simulink library "halout"  (R2021b)
settings: Solver=VariableStepAuto  StartTime=0.0  StopTime=10.0  RelTol=1e-3
undefined symbols (not defined in the file): C_TASK_5MS_S, FALSE, KHAL_CAN1FDAPS3E2E_flg, KHAL_CAN1FDAPS3TxReq_flg, KHAL_CAN1FDVCU2E2E_flg, KHAL_CAN1FDVCU2TxReq_flg, KHAL_CAN1FDVCU3E2E_flg, KHAL_CAN1FDVCU3TxReq_flg, KHAL_CAN1TxReq_flg, KHAL_CAN2TxReq_flg, KHAL_CAN3FDVCU1TxReq_flg, KHAL_CAN3FDVCU2E2E_flg, KHAL_CAN3FDVCU2TxReq_flg, KHAL_CAN3TxReq_flg, KHAL_CAN4FDVCU1E2E_flg, KHAL_CAN4FDVCU1TxReq_flg, KHAL_CAN4TxReq_flg, KHAL_CAN5TxReq_flg, ONE_INT, TRUE, ZERO_INT
libraries: FVT_lib x383, simulink x179
(part 18 of 20)

== system halout/HAL_OUT/CAN4/FD_THCM2_0x186/FDEXV2Cmd ==
  FDEXV2Cmd : Inport
  Data Type Conversion : DataTypeConversion  OutDataTypeStr=uint16  RndMeth=Round
  CAN4_FD_EXV2_Cmd : Outport
  wires:
  Data Type Conversion/1 -> CAN4_FD_EXV2_Cmd/1
  FDEXV2Cmd/1 -> Data Type Conversion/1

== system halout/HAL_OUT/CAN4/FD_THCM2_0x186/FDFWVCmd ==
  FDFWVCmd : Inport
  Data Type Conversion : DataTypeConversion  OutDataTypeStr=uint8  RndMeth=Round
  CAN4_FD_FWV_Cmd : Outport
  wires:
  Data Type Conversion/1 -> CAN4_FD_FWV_Cmd/1
  FDFWVCmd/1 -> Data Type Conversion/1

== system halout/HAL_OUT/CAN4/FD_THCM2_0x186/FDFrLeAPTCHeatPwrCmd ==
  FDFrLeAPTCHeatPwrCmd : Inport
  Data Type Conversion : DataTypeConversion  OutDataTypeStr=uint8  RndMeth=Round
  convert_out : FVT_lib/hal/convert_out  gain=25  offset=0
  CAN4_FD_FrLeAPTCHeatPwr_Cmd : Outport
  wires:
  Data Type Conversion/1 -> CAN4_FD_FrLeAPTCHeatPwr_Cmd/1
  convert_out/1 -> Data Type Conversion/1
  FDFrLeAPTCHeatPwrCmd/1 -> convert_out/1

== system halout/HAL_OUT/CAN4/FD_THCM2_0x186/FDFrRiAPTCHeatPwrCmd ==
  FDFrRiAPTCHeatPwrCmd : Inport
  Data Type Conversion : DataTypeConversion  OutDataTypeStr=uint8  RndMeth=Round
  convert_out : FVT_lib/hal/convert_out  gain=25  offset=0
  CAN4_FD_FrRiAPTCHeatPwr_Cmd : Outport
  wires:
  Data Type Conversion/1 -> CAN4_FD_FrRiAPTCHeatPwr_Cmd/1
  convert_out/1 -> Data Type Conversion/1
  FDFrRiAPTCHeatPwrCmd/1 -> convert_out/1

== system halout/HAL_OUT/CAN4/FD_THCM2_0x186/FDFrWPTCHeatPwrCmd ==
  FDFrWPTCHeatPwrCmd : Inport
  Data Type Conversion : DataTypeConversion  OutDataTypeStr=uint16  RndMeth=Round
  CAN4_FD_FrWPTCHeatPwr_Cmd : Outport
  wires:
  Data Type Conversion/1 -> CAN4_FD_FrWPTCHeatPwr_Cmd/1
  FDFrWPTCHeatPwrCmd/1 -> Data Type Conversion/1

== system halout/HAL_OUT/CAN4/FD_THCM2_0x186/FDRrAPTCHeatPwrCmd ==
  FDRrAPTCHeatPwrCmd : Inport
  Data Type Conversion : DataTypeConversion  OutDataTypeStr=uint8  RndMeth=Round
  convert_out : FVT_lib/hal/convert_out  gain=25  offset=0
  CAN4_FD_RrAPTCHeatPwr_Cmd : Outport
  wires:
  Data Type Conversion/1 -> CAN4_FD_RrAPTCHeatPwr_Cmd/1
  convert_out/1 -> Data Type Conversion/1
  FDRrAPTCHeatPwrCmd/1 -> convert_out/1

== system halout/HAL_OUT/CAN4/FD_THCM2_0x186/FDSOTXVCmd ==
  FDSOTXVCmd : Inport
  Data Type Conversion : DataTypeConversion  OutDataTypeStr=uint8  RndMeth=Round
  CAN4_FD_SOTXV_Cmd : Outport
  wires:
  Data Type Conversion/1 -> CAN4_FD_SOTXV_Cmd/1
  FDSOTXVCmd/1 -> Data Type Conversion/1

== system halout/HAL_OUT/CAN4/FD_THCM2_0x186/FDSOV1Cmd ==
  FDSOV1Cmd : Inport
  Data Type Conversion : DataTypeConversion  OutDataTypeStr=uint8  RndMeth=Round
  CAN4_FD_SOV1_Cmd : Outport
  wires:
  Data Type Conversion/1 -> CAN4_FD_SOV1_Cmd/1
  FDSOV1Cmd/1 -> Data Type Conversion/1

== system halout/HAL_OUT/CAN4/FD_THCM2_0x186/FDSOV2Cmd ==
  FDSOV2Cmd : Inport
  Data Type Conversion : DataTypeConversion  OutDataTypeStr=uint8  RndMeth=Round
  CAN4_FD_SOV2_Cmd : Outport
  wires:
  Data Type Conversion/1 -> CAN4_FD_SOV2_Cmd/1
  FDSOV2Cmd/1 -> Data Type Conversion/1

== system halout/HAL_OUT/CAN4/FD_THCM2_0x186/FDSOV3Cmd ==
  FDSOV3Cmd : Inport
  Data Type Conversion : DataTypeConversion  OutDataTypeStr=uint8  RndMeth=Round
  CAN4_FD_SOV3_Cmd : Outport
  wires:
  Data Type Conversion/1 -> CAN4_FD_SOV3_Cmd/1
  FDSOV3Cmd/1 -> Data Type Conversion/1

== system halout/HAL_OUT/CAN4/FD_THCM2_0x186/FDTWVCmd ==
  FDTWVCmd : Inport
  Data Type Conversion : DataTypeConversion  OutDataTypeStr=uint8  RndMeth=Round
  convert_out : FVT_lib/hal/convert_out  gain=0.392  offset=0
  CAN4_FD_TWV_Cmd : Outport
  wires:
  Data Type Conversion/1 -> CAN4_FD_TWV_Cmd/1
  convert_out/1 -> Data Type Conversion/1
  FDTWVCmd/1 -> convert_out/1

== system halout/HAL_OUT/CAN4/FD_VCU1_0x116/AllDoorSW ==
  AllDoorSW : Inport
  Data Type Conversion : DataTypeConversion  OutDataTypeStr=uint8  RndMeth=Round
  CAN4_AllDoorSW : Outport
  wires:
  Data Type Conversion/1 -> CAN4_AllDoorSW/1
  AllDoorSW/1 -> Data Type Conversion/1

== system halout/HAL_OUT/CAN4/FD_VCU1_0x116/AmbLightBreath1 ==
  AmbLightBreath1 : Inport
  Data Type Conversion : DataTypeConversion  OutDataTypeStr=uint8  RndMeth=Round
  CAN4_AmbLightBreath1 : Outport
  wires:
  Data Type Conversion/1 -> CAN4_AmbLightBreath1/1
  AmbLightBreath1/1 -> Data Type Conversion/1

== system halout/HAL_OUT/CAN4/FD_VCU1_0x116/AmbLightBreath2 ==
  AmbLightBreath2 : Inport
  Data Type Conversion : DataTypeConversion  OutDataTypeStr=uint8  RndMeth=Round
  CAN4_AmbLightBreath2 : Outport
  wires:
  Data Type Conversion/1 -> CAN4_AmbLightBreath2/1
  AmbLightBreath2/1 -> Data Type Conversion/1

== system halout/HAL_OUT/CAN4/FD_VCU1_0x116/AmbLightBreath3 ==
  AmbLightBreath3 : Inport
  Data Type Conversion : DataTypeConversion  OutDataTypeStr=uint8  RndMeth=Round
  CAN4_AmbLightBreath3 : Outport
  wires:
  Data Type Conversion/1 -> CAN4_AmbLightBreath3/1
  AmbLightBreath3/1 -> Data Type Conversion/1

== system halout/HAL_OUT/CAN4/FD_VCU1_0x116/AmbLightBrightness1 ==
  AmbLightBrightness1 : Inport
  Data Type Conversion : DataTypeConversion  OutDataTypeStr=uint8  RndMeth=Round
  CAN4_AmbLightBrightness1 : Outport
  wires:
  Data Type Conversion/1 -> CAN4_AmbLightBrightness1/1
  AmbLightBrightness1/1 -> Data Type Conversion/1

== system halout/HAL_OUT/CAN4/FD_VCU1_0x116/AmbLightBrightness2 ==
  AmbLightBrightness2 : Inport
  Data Type Conversion : DataTypeConversion  OutDataTypeStr=uint8  RndMeth=Round
  CAN4_AmbLightBrightness2 : Outport
  wires:
  Data Type Conversion/1 -> CAN4_AmbLightBrightness2/1
  AmbLightBrightness2/1 -> Data Type Conversion/1

== system halout/HAL_OUT/CAN4/FD_VCU1_0x116/AmbLightBrightness3 ==
  AmbLightBrightness3 : Inport
  Data Type Conversion : DataTypeConversion  OutDataTypeStr=uint8  RndMeth=Round
  CAN4_AmbLightBrightness3 : Outport
  wires:
  Data Type Conversion/1 -> CAN4_AmbLightBrightness3/1
  AmbLightBrightness3/1 -> Data Type Conversion/1

== system halout/HAL_OUT/CAN4/FD_VCU1_0x116/AmbLightColor1 ==
  AmbLightColor1 : Inport
  Data Type Conversion : DataTypeConversion  OutDataTypeStr=uint8  RndMeth=Round
  CAN4_AmbLightColor1 : Outport
  wires:
  Data Type Conversion/1 -> CAN4_AmbLightColor1/1
  AmbLightColor1/1 -> Data Type Conversion/1

== system halout/HAL_OUT/CAN4/FD_VCU1_0x116/AmbLightColor2 ==
  AmbLightColor2 : Inport
  Data Type Conversion : DataTypeConversion  OutDataTypeStr=uint8  RndMeth=Round
  CAN4_AmbLightColor2 : Outport
  wires:
  Data Type Conversion/1 -> CAN4_AmbLightColor2/1
  AmbLightColor2/1 -> Data Type Conversion/1

== system halout/HAL_OUT/CAN4/FD_VCU1_0x116/AmbLightColor3 ==
  AmbLightColor3 : Inport
  Data Type Conversion : DataTypeConversion  OutDataTypeStr=uint8  RndMeth=Round
  CAN4_AmbLightColor3 : Outport
  wires:
  Data Type Conversion/1 -> CAN4_AmbLightColor3/1
  AmbLightColor3/1 -> Data Type Conversion/1

== system halout/HAL_OUT/CAN4/FD_VCU1_0x116/AntiTheftSeatFold ==
  AntiTheftSeatFold : Inport
  Data Type Conversion : DataTypeConversion  OutDataTypeStr=uint8  RndMeth=Round
  CAN4_AntiTheftSeatFold : Outport
  wires:
  Data Type Conversion/1 -> CAN4_AntiTheftSeatFold/1
  AntiTheftSeatFold/1 -> Data Type Conversion/1

== system halout/HAL_OUT/CAN4/FD_VCU1_0x116/AntitheftSta ==
  AntitheftSta : Inport
  Data Type Conversion : DataTypeConversion  OutDataTypeStr=uint8  RndMeth=Round
  CAN4_AntitheftSta : Outport
  wires:
  Data Type Conversion/1 -> CAN4_AntitheftSta/1
  AntitheftSta/1 -> Data Type Conversion/1

== system halout/HAL_OUT/CAN4/FD_VCU1_0x116/BCMBuzzerReq ==
  BCMBuzzerReq : Inport
  Data Type Conversion : DataTypeConversion  OutDataTypeStr=uint8  RndMeth=Round
  CAN4_BCM_Buzzer_Req : Outport
  wires:
  Data Type Conversion/1 -> CAN4_BCM_Buzzer_Req/1
  BCMBuzzerReq/1 -> Data Type Conversion/1

== system halout/HAL_OUT/CAN4/FD_VCU1_0x116/BCMDoorLockSta ==
  BCMDoorLockSta : Inport
  Data Type Conversion : DataTypeConversion  OutDataTypeStr=uint8  RndMeth=Round
  CAN4_BCM_DoorLock_Sta : Outport
  wires:
  Data Type Conversion/1 -> CAN4_BCM_DoorLock_Sta/1
  BCMDoorLockSta/1 -> Data Type Conversion/1

== system halout/HAL_OUT/CAN4/FD_VCU1_0x116/BrakeLamp ==
  BrakeLamp : Inport
  Data Type Conversion : DataTypeConversion  OutDataTypeStr=uint8  RndMeth=Round
  CAN4_BrakeLamp : Outport
  wires:
  Data Type Conversion/1 -> CAN4_BrakeLamp/1
  BrakeLamp/1 -> Data Type Conversion/1

== system halout/HAL_OUT/CAN4/FD_VCU1_0x116/Byte_0 ==
  CS_VCU1_CAN4 : Inport
  BitwiseOR : simulink/Logic and Bit Operations/Bitwise Operator  logicop=OR  UseBitMask=off  BitMask=bin2dec('11011001')  BitMaskRealWorld=Stored Integer
  SignalPack : FVT_lib/hal/SignalPack  RightShiftCnt=0  BitMask=2^8-1  LeftShiftCnt=0
  UnitConverter : DataTypeConversion  OutDataTypeStr=uint8  RndMeth=Round
  UnitConverter1 : DataTypeConversion  OutDataTypeStr=uint8  RndMeth=Round
  Byte_0 : Outport
  wires:
  BitwiseOR/1 -> Byte_0/1
  UnitConverter/1 -> BitwiseOR/1
  SignalPack/1 -> UnitConverter/1
  UnitConverter1/1 -> SignalPack/1
  CS_VCU1_CAN4/1 -> UnitConverter1/1

== system halout/HAL_OUT/CAN4/FD_VCU1_0x116/Byte_1 ==
  RC_VCU1_CAN4 : Inport
  BitwiseOR : simulink/Logic and Bit Operations/Bitwise Operator  logicop=OR  UseBitMask=off  BitMask=bin2dec('11011001')  BitMaskRealWorld=Stored Integer
  SignalPack : FVT_lib/hal/SignalPack  RightShiftCnt=0  BitMask=2^4-1  LeftShiftCnt=0
  UnitConverter : DataTypeConversion  OutDataTypeStr=uint8  RndMeth=Round
  UnitConverter1 : DataTypeConversion  OutDataTypeStr=uint8  RndMeth=Round
  Byte_1 : Outport
  wires:
  BitwiseOR/1 -> Byte_1/1
  UnitConverter/1 -> BitwiseOR/1
  SignalPack/1 -> UnitConverter/1
  UnitConverter1/1 -> SignalPack/1
  RC_VCU1_CAN4/1 -> UnitConverter1/1

== system halout/HAL_OUT/CAN4/FD_VCU1_0x116/Byte_10 ==
  TimeSNDKCFbk : Inport
  BitwiseOR : simulink/Logic and Bit Operations/Bitwise Operator  logicop=OR  UseBitMask=off  BitMask=bin2dec('11011001')  BitMaskRealWorld=Stored Integer
  SignalPack : FVT_lib/hal/SignalPack  RightShiftCnt=8  BitMask=2^8-1  LeftShiftCnt=0
  UnitConverter : DataTypeConversion  OutDataTypeStr=uint8  RndMeth=Round
  UnitConverter1 : DataTypeConversion  OutDataTypeStr=uint32  RndMeth=Round
  Byte_10 : Outport
  wires:
  BitwiseOR/1 -> Byte_10/1
  UnitConverter/1 -> BitwiseOR/1
  SignalPack/1 -> UnitConverter/1
  UnitConverter1/1 -> SignalPack/1
  TimeSNDKCFbk/1 -> UnitConverter1/1

== system halout/HAL_OUT/CAN4/FD_VCU1_0x116/Byte_11 ==
  TimeSNDKCFbk : Inport
  BitwiseOR : simulink/Logic and Bit Operations/Bitwise Operator  logicop=OR  UseBitMask=off  BitMask=bin2dec('11011001')  BitMaskRealWorld=Stored Integer
  SignalPack : FVT_lib/hal/SignalPack  RightShiftCnt=0  BitMask=2^8-1  LeftShiftCnt=0
  UnitConverter : DataTypeConversion  OutDataTypeStr=uint8  RndMeth=Round
  UnitConverter1 : DataTypeConversion  OutDataTypeStr=uint32  RndMeth=Round
  Byte_11 : Outport
  wires:
  BitwiseOR/1 -> Byte_11/1
  UnitConverter/1 -> BitwiseOR/1
  SignalPack/1 -> UnitConverter/1
  UnitConverter1/1 -> SignalPack/1
  TimeSNDKCFbk/1 -> UnitConverter1/1

== system halout/HAL_OUT/CAN4/FD_VCU1_0x116/Byte_12 ==
  BCM_DoorLock_Sta : Inport
  DimmerEN : Inport  Port=2
  EquivAccPedalSWSta : Inport  Port=3
  HornCtrl : Inport  Port=4
  RoomLampH : Inport  Port=5
  RoomLampL : Inport  Port=6
  TailgateRemote : Inport  Port=7
  BitwiseOR : simulink/Logic and Bit Operations/Bitwise Operator  logicop=OR  UseBitMask=off  NumInputPorts=7  BitMask=bin2dec('11011001')  BitMaskRealWorld=Stored Integer
  SignalPack : FVT_lib/hal/SignalPack  RightShiftCnt=0  BitMask=2^1-1  LeftShiftCnt=4
  SignalPack1 : FVT_lib/hal/SignalPack  RightShiftCnt=0  BitMask=2^1-1  LeftShiftCnt=3
  SignalPack2 : FVT_lib/hal/SignalPack  RightShiftCnt=0  BitMask=2^1-1  LeftShiftCnt=6
  SignalPack3 : FVT_lib/hal/SignalPack  RightShiftCnt=0  BitMask=2^1-1  LeftShiftCnt=5
  SignalPack4 : FVT_lib/hal/SignalPack  RightShiftCnt=0  BitMask=2^1-1  LeftShiftCnt=2
  SignalPack5 : FVT_lib/hal/SignalPack  RightShiftCnt=0  BitMask=2^1-1  LeftShiftCnt=1
  SignalPack6 : FVT_lib/hal/SignalPack  RightShiftCnt=1  BitMask=2^1-1  LeftShiftCnt=0
  UnitConverter{,1..13} (14 alike) : DataTypeConversion  OutDataTypeStr=uint8  RndMeth=Round
  Byte_12 : Outport
  wires:
  BitwiseOR/1 -> Byte_12/1
  UnitConverter/1 -> BitwiseOR/1
  SignalPack/1 -> UnitConverter/1
  UnitConverter1/1 -> SignalPack/1
  BCM_DoorLock_Sta/1 -> UnitConverter1/1
  UnitConverter2/1 -> BitwiseOR/2
  SignalPack1/1 -> UnitConverter2/1
  UnitConverter3/1 -> SignalPack1/1
  DimmerEN/1 -> UnitConverter3/1
  UnitConverter4/1 -> BitwiseOR/3
  SignalPack2/1 -> UnitConverter4/1
  UnitConverter5/1 -> SignalPack2/1
  EquivAccPedalSWSta/1 -> UnitConverter5/1
  UnitConverter6/1 -> BitwiseOR/4
  SignalPack3/1 -> UnitConverter6/1
  UnitConverter7/1 -> SignalPack3/1
  HornCtrl/1 -> UnitConverter7/1
  UnitConverter8/1 -> BitwiseOR/5
  SignalPack4/1 -> UnitConverter8/1
  UnitConverter9/1 -> SignalPack4/1
  RoomLampH/1 -> UnitConverter9/1
  UnitConverter10/1 -> BitwiseOR/6
  SignalPack5/1 -> UnitConverter10/1
  UnitConverter11/1 -> SignalPack5/1
  RoomLampL/1 -> UnitConverter11/1
  UnitConverter12/1 -> BitwiseOR/7
  SignalPack6/1 -> UnitConverter12/1
  UnitConverter13/1 -> SignalPack6/1
  TailgateRemote/1 -> UnitConverter13/1

== system halout/HAL_OUT/CAN4/FD_VCU1_0x116/Byte_13 ==
  BCM_Buzzer_Req : Inport
  Dimmer : Inport  Port=2
  LockSetting : Inport  Port=3
  TailgateRemote : Inport  Port=4
  BitwiseOR : simulink/Logic and Bit Operations/Bitwise Operator  logicop=OR  UseBitMask=off  NumInputPorts=4  BitMask=bin2dec('11011001')  BitMaskRealWorld=Stored Integer
  SignalPack : FVT_lib/hal/SignalPack  RightShiftCnt=0  BitMask=2^1-1  LeftShiftCnt=6
  SignalPack1 : FVT_lib/hal/SignalPack  RightShiftCnt=2  BitMask=2^5-1  LeftShiftCnt=0
  SignalPack2 : FVT_lib/hal/SignalPack  RightShiftCnt=0  BitMask=2^1-1  LeftShiftCnt=5
  SignalPack3 : FVT_lib/hal/SignalPack  RightShiftCnt=0  BitMask=2^1-1  LeftShiftCnt=7
  UnitConverter{,1..7} (8 alike) : DataTypeConversion  OutDataTypeStr=uint8  RndMeth=Round
  Byte_13 : Outport
  wires:
  BitwiseOR/1 -> Byte_13/1
  UnitConverter/1 -> BitwiseOR/1
  SignalPack/1 -> UnitConverter/1
  UnitConverter1/1 -> SignalPack/1
  BCM_Buzzer_Req/1 -> UnitConverter1/1
  UnitConverter2/1 -> BitwiseOR/2
  SignalPack1/1 -> UnitConverter2/1
  UnitConverter3/1 -> SignalPack1/1
  Dimmer/1 -> UnitConverter3/1
  UnitConverter4/1 -> BitwiseOR/3
  SignalPack2/1 -> UnitConverter4/1
  UnitConverter5/1 -> SignalPack2/1
  LockSetting/1 -> UnitConverter5/1
  UnitConverter6/1 -> BitwiseOR/4
  SignalPack3/1 -> UnitConverter6/1
  UnitConverter7/1 -> SignalPack3/1
  TailgateRemote/1 -> UnitConverter7/1

== system halout/HAL_OUT/CAN4/FD_VCU1_0x116/Byte_14 ==
  AntiTheftSeatFold : Inport
  AntitheftSta : Inport  Port=2
  CrashDetd : Inport  Port=3
  Dimmer : Inport  Port=4
  L_APM_WdwEnable : Inport  Port=5
  RTurnLP : Inport  Port=6
  BitwiseOR : simulink/Logic and Bit Operations/Bitwise Operator  logicop=OR  UseBitMask=off  NumInputPorts=6  BitMask=bin2dec('11011001')  BitMaskRealWorld=Stored Integer
  SignalPack : FVT_lib/hal/SignalPack  RightShiftCnt=0  BitMask=2^1-1  LeftShiftCnt=3
  SignalPack1 : FVT_lib/hal/SignalPack  RightShiftCnt=0  BitMask=2^2-1  LeftShiftCnt=1
  SignalPack2 : FVT_lib/hal/SignalPack  RightShiftCnt=0  BitMask=2^1-1  LeftShiftCnt=4
  SignalPack3 : FVT_lib/hal/SignalPack  RightShiftCnt=0  BitMask=2^2-1  LeftShiftCnt=6
  SignalPack4 : FVT_lib/hal/SignalPack  RightShiftCnt=0  BitMask=2^1-1  LeftShiftCnt=5
  SignalPack5 : FVT_lib/hal/SignalPack  RightShiftCnt=0  BitMask=2^1-1  LeftShiftCnt=0
  UnitConverter{,1..11} (12 alike) : DataTypeConversion  OutDataTypeStr=uint8  RndMeth=Round
  Byte_14 : Outport
  wires:
  BitwiseOR/1 -> Byte_14/1
  UnitConverter/1 -> BitwiseOR/1
  SignalPack/1 -> UnitConverter/1
  UnitConverter1/1 -> SignalPack/1
  AntiTheftSeatFold/1 -> UnitConverter1/1
  UnitConverter2/1 -> BitwiseOR/2
  SignalPack1/1 -> UnitConverter2/1
  UnitConverter3/1 -> SignalPack1/1
  AntitheftSta/1 -> UnitConverter3/1
  UnitConverter4/1 -> BitwiseOR/3
  SignalPack2/1 -> UnitConverter4/1
  UnitConverter5/1 -> SignalPack2/1
  CrashDetd/1 -> UnitConverter5/1
  UnitConverter6/1 -> BitwiseOR/4
  SignalPack3/1 -> UnitConverter6/1
  UnitConverter7/1 -> SignalPack3/1
  Dimmer/1 -> UnitConverter7/1
  UnitConverter8/1 -> BitwiseOR/5
  SignalPack4/1 -> UnitConverter8/1
  UnitConverter9/1 -> SignalPack4/1
  L_APM_WdwEnable/1 -> UnitConverter9/1
  UnitConverter10/1 -> BitwiseOR/6
  SignalPack5/1 -> UnitConverter10/1
  UnitConverter11/1 -> SignalPack5/1
  RTurnLP/1 -> UnitConverter11/1

== system halout/HAL_OUT/CAN4/FD_VCU1_0x116/Byte_15 ==
  BrakeLamp : Inport
  Fr_FogLamp : Inport  Port=2
  HazardSW : Inport  Port=3
  LBSD : Inport  Port=4
  LTurnLP : Inport  Port=5
  RBSD : Inport  Port=6
  ReverseLamp : Inport  Port=7
  Rr_FogLamp : Inport  Port=8
  BitwiseOR : simulink/Logic and Bit Operations/Bitwise Operator  logicop=OR  UseBitMask=off  NumInputPorts=8  BitMask=bin2dec('11011001')  BitMaskRealWorld=Stored Integer
  SignalPack : FVT_lib/hal/SignalPack  RightShiftCnt=0  BitMask=2^1-1  LeftShiftCnt=1
  SignalPack1 : FVT_lib/hal/SignalPack  RightShiftCnt=0  BitMask=2^1-1  LeftShiftCnt=4
  SignalPack2 : FVT_lib/hal/SignalPack  RightShiftCnt=0  BitMask=2^1-1  LeftShiftCnt=6
  SignalPack3 : FVT_lib/hal/SignalPack  RightShiftCnt=0  BitMask=2^1-1  LeftShiftCnt=2
  SignalPack4 : FVT_lib/hal/SignalPack  RightShiftCnt=0  BitMask=2^1-1  LeftShiftCnt=7
  SignalPack5 : FVT_lib/hal/SignalPack  RightShiftCnt=0  BitMask=2^1-1  LeftShiftCnt=3
  SignalPack6 : FVT_lib/hal/SignalPack  RightShiftCnt=0  BitMask=2^1-1  LeftShiftCnt=0
  SignalPack7 : FVT_lib/hal/SignalPack  RightShiftCnt=0  BitMask=2^1-1  LeftShiftCnt=5
  UnitConverter{,1..15} (16 alike) : DataTypeConversion  OutDataTypeStr=uint8  RndMeth=Round
  Byte_15 : Outport
  wires:
  BitwiseOR/1 -> Byte_15/1
  UnitConverter/1 -> BitwiseOR/1
  SignalPack/1 -> UnitConverter/1
  UnitConverter1/1 -> SignalPack/1
  BrakeLamp/1 -> UnitConverter1/1
  UnitConverter2/1 -> BitwiseOR/2
  SignalPack1/1 -> UnitConverter2/1
  UnitConverter3/1 -> SignalPack1/1
  Fr_FogLamp/1 -> UnitConverter3/1
  UnitConverter4/1 -> BitwiseOR/3
  SignalPack2/1 -> UnitConverter4/1
  UnitConverter5/1 -> SignalPack2/1
  HazardSW/1 -> UnitConverter5/1
  UnitConverter6/1 -> BitwiseOR/4
  SignalPack3/1 -> UnitConverter6/1
  UnitConverter7/1 -> SignalPack3/1
  LBSD/1 -> UnitConverter7/1
  UnitConverter8/1 -> BitwiseOR/5
  SignalPack4/1 -> UnitConverter8/1
  UnitConverter9/1 -> SignalPack4/1
  LTurnLP/1 -> UnitConverter9/1
  UnitConverter10/1 -> BitwiseOR/6
  SignalPack5/1 -> UnitConverter10/1
  UnitConverter11/1 -> SignalPack5/1
  RBSD/1 -> UnitConverter11/1
  UnitConverter12/1 -> BitwiseOR/7
  SignalPack6/1 -> UnitConverter12/1
  UnitConverter13/1 -> SignalPack6/1
  ReverseLamp/1 -> UnitConverter13/1
  UnitConverter14/1 -> BitwiseOR/8
  SignalPack7/1 -> UnitConverter14/1
  UnitConverter15/1 -> SignalPack7/1
  Rr_FogLamp/1 -> UnitConverter15/1

== system halout/HAL_OUT/CAN4/FD_VCU1_0x116/Byte_16 ==
  H_Beam : Inport
  LDRL : Inport  Port=2
  L_Beam : Inport  Port=3
  PosLamp : Inport  Port=4
  RDRL : Inport  Port=5
  WasherCtrl : Inport  Port=6
  WiperFixMode : Inport  Port=7
  BitwiseOR : simulink/Logic and Bit Operations/Bitwise Operator  logicop=OR  UseBitMask=off  NumInputPorts=7  BitMask=bin2dec('11011001')  BitMaskRealWorld=Stored Integer
  SignalPack : FVT_lib/hal/SignalPack  RightShiftCnt=0  BitMask=2^1-1  LeftShiftCnt=4
  SignalPack1 : FVT_lib/hal/SignalPack  RightShiftCnt=0  BitMask=2^1-1  LeftShiftCnt=6
  SignalPack2 : FVT_lib/hal/SignalPack  RightShiftCnt=0  BitMask=2^1-1  LeftShiftCnt=3
  SignalPack3 : FVT_lib/hal/SignalPack  RightShiftCnt=0  BitMask=2^1-1  LeftShiftCnt=5
  SignalPack4 : FVT_lib/hal/SignalPack  RightShiftCnt=0  BitMask=2^1-1  LeftShiftCnt=7
  SignalPack5 : FVT_lib/hal/SignalPack  RightShiftCnt=0  BitMask=2^2-1  LeftShiftCnt=1
  SignalPack6 : FVT_lib/hal/SignalPack  RightShiftCnt=0  BitMask=2^1-1  LeftShiftCnt=0
  UnitConverter{,1..13} (14 alike) : DataTypeConversion  OutDataTypeStr=uint8  RndMeth=Round
  Byte_16 : Outport
  wires:
  BitwiseOR/1 -> Byte_16/1
  UnitConverter/1 -> BitwiseOR/1
  SignalPack/1 -> UnitConverter/1
  UnitConverter1/1 -> SignalPack/1
  H_Beam/1 -> UnitConverter1/1
  UnitConverter2/1 -> BitwiseOR/2
  SignalPack1/1 -> UnitConverter2/1
  UnitConverter3/1 -> SignalPack1/1
  LDRL/1 -> UnitConverter3/1
  UnitConverter4/1 -> BitwiseOR/3
  SignalPack2/1 -> UnitConverter4/1
  UnitConverter5/1 -> SignalPack2/1
  L_Beam/1 -> UnitConverter5/1
  UnitConverter6/1 -> BitwiseOR/4
  SignalPack3/1 -> UnitConverter6/1
  UnitConverter7/1 -> SignalPack3/1
  PosLamp/1 -> UnitConverter7/1
  UnitConverter8/1 -> BitwiseOR/5
  SignalPack4/1 -> UnitConverter8/1
  UnitConverter9/1 -> SignalPack4/1
  RDRL/1 -> UnitConverter9/1
  UnitConverter10/1 -> BitwiseOR/6
  SignalPack5/1 -> UnitConverter10/1
  UnitConverter11/1 -> SignalPack5/1
  WasherCtrl/1 -> UnitConverter11/1
  UnitConverter12/1 -> BitwiseOR/7
  SignalPack6/1 -> UnitConverter12/1
  UnitConverter13/1 -> SignalPack6/1
  WiperFixMode/1 -> UnitConverter13/1

== system halout/HAL_OUT/CAN4/FD_VCU1_0x116/Byte_17 ==
  Fr_Wiper_H : Inport
  Fr_Wiper_L : Inport  Port=2
  MirrorCtrl : Inport  Port=3
  Rr_Defog : Inport  Port=4
  Rr_Wiper : Inport  Port=5
  TailgateHDSW : Inport  Port=6
  TrunkRel : Inport  Port=7
  BitwiseOR : simulink/Logic and Bit Operations/Bitwise Operator  logicop=OR  UseBitMask=off  NumInputPorts=7  BitMask=bin2dec('11011001')  BitMaskRealWorld=Stored Integer
  SignalPack : FVT_lib/hal/SignalPack  RightShiftCnt=0  BitMask=2^1-1  LeftShiftCnt=5
  SignalPack1 : FVT_lib/hal/SignalPack  RightShiftCnt=0  BitMask=2^1-1  LeftShiftCnt=6
  SignalPack2 : FVT_lib/hal/SignalPack  RightShiftCnt=0  BitMask=2^2-1  LeftShiftCnt=3
  SignalPack3 : FVT_lib/hal/SignalPack  RightShiftCnt=0  BitMask=2^1-1  LeftShiftCnt=0
  SignalPack4 : FVT_lib/hal/SignalPack  RightShiftCnt=0  BitMask=2^1-1  LeftShiftCnt=7
  SignalPack5 : FVT_lib/hal/SignalPack  RightShiftCnt=0  BitMask=2^1-1  LeftShiftCnt=2
  SignalPack6 : FVT_lib/hal/SignalPack  RightShiftCnt=0  BitMask=2^1-1  LeftShiftCnt=1
  UnitConverter{,1..13} (14 alike) : DataTypeConversion  OutDataTypeStr=uint8  RndMeth=Round
  Byte_17 : Outport
  wires:
  BitwiseOR/1 -> Byte_17/1
  UnitConverter/1 -> BitwiseOR/1
  SignalPack/1 -> UnitConverter/1
  UnitConverter1/1 -> SignalPack/1
  Fr_Wiper_H/1 -> UnitConverter1/1
  UnitConverter2/1 -> BitwiseOR/2
  SignalPack1/1 -> UnitConverter2/1
  UnitConverter3/1 -> SignalPack1/1
  Fr_Wiper_L/1 -> UnitConverter3/1
  UnitConverter4/1 -> BitwiseOR/3
  SignalPack2/1 -> UnitConverter4/1
  UnitConverter5/1 -> SignalPack2/1
  MirrorCtrl/1 -> UnitConverter5/1
  UnitConverter6/1 -> BitwiseOR/4
  SignalPack3/1 -> UnitConverter6/1
  UnitConverter7/1 -> SignalPack3/1
  Rr_Defog/1 -> UnitConverter7/1
  UnitConverter8/1 -> BitwiseOR/5
  SignalPack4/1 -> UnitConverter8/1
  UnitConverter9/1 -> SignalPack4/1
  Rr_Wiper/1 -> UnitConverter9/1
  UnitConverter10/1 -> BitwiseOR/6
  SignalPack5/1 -> UnitConverter10/1
  UnitConverter11/1 -> SignalPack5/1
  TailgateHDSW/1 -> UnitConverter11/1
  UnitConverter12/1 -> BitwiseOR/7
  SignalPack6/1 -> UnitConverter12/1
  UnitConverter13/1 -> SignalPack6/1
  TrunkRel/1 -> UnitConverter13/1

== system halout/HAL_OUT/CAN4/FD_VCU1_0x116/Byte_18 ==
  CTDCtrl : Inport
  CTDLockSW : Inport  Port=2
  CTDUnlockSW : Inport  Port=3
  Fr_ChargingDoorCtrl : Inport  Port=4
  MirrorDefog : Inport  Port=5
  Rr_ChargingDoorCtrl : Inport  Port=6
  BitwiseOR : simulink/Logic and Bit Operations/Bitwise Operator  logicop=OR  UseBitMask=off  NumInputPorts=6  BitMask=bin2dec('11011001')  BitMaskRealWorld=Stored Integer
  SignalPack : FVT_lib/hal/SignalPack  RightShiftCnt=1  BitMask=2^1-1  LeftShiftCnt=0
  SignalPack1 : FVT_lib/hal/SignalPack  RightShiftCnt=0  BitMask=2^1-1  LeftShiftCnt=5
  SignalPack2 : FVT_lib/hal/SignalPack  RightShiftCnt=0  BitMask=2^1-1  LeftShiftCnt=6
  SignalPack3 : FVT_lib/hal/SignalPack  RightShiftCnt=0  BitMask=2^2-1  LeftShiftCnt=1
  SignalPack4 : FVT_lib/hal/SignalPack  RightShiftCnt=0  BitMask=2^1-1  LeftShiftCnt=7
  SignalPack5 : FVT_lib/hal/SignalPack  RightShiftCnt=0  BitMask=2^2-1  LeftShiftCnt=3
  UnitConverter{,1..11} (12 alike) : DataTypeConversion  OutDataTypeStr=uint8  RndMeth=Round
  Byte_18 : Outport
  wires:
  BitwiseOR/1 -> Byte_18/1
  UnitConverter/1 -> BitwiseOR/1
  SignalPack/1 -> UnitConverter/1
  UnitConverter1/1 -> SignalPack/1
  CTDCtrl/1 -> UnitConverter1/1
  UnitConverter2/1 -> BitwiseOR/2
  SignalPack1/1 -> UnitConverter2/1
  UnitConverter3/1 -> SignalPack1/1
  CTDLockSW/1 -> UnitConverter3/1
  UnitConverter4/1 -> BitwiseOR/3
  SignalPack2/1 -> UnitConverter4/1
  UnitConverter5/1 -> SignalPack2/1
  CTDUnlockSW/1 -> UnitConverter5/1
  UnitConverter6/1 -> BitwiseOR/4
  SignalPack3/1 -> UnitConverter6/1
  UnitConverter7/1 -> SignalPack3/1
  Fr_ChargingDoorCtrl/1 -> UnitConverter7/1
  UnitConverter8/1 -> BitwiseOR/5
  SignalPack4/1 -> UnitConverter8/1
  UnitConverter9/1 -> SignalPack4/1
  MirrorDefog/1 -> UnitConverter9/1
  UnitConverter10/1 -> BitwiseOR/6
  SignalPack5/1 -> UnitConverter10/1
  UnitConverter11/1 -> SignalPack5/1
  Rr_ChargingDoorCtrl/1 -> UnitConverter11/1

== system halout/HAL_OUT/CAN4/FD_VCU1_0x116/Byte_19 ==
  AllDoorSW : Inport
  CTDCtrl : Inport  Port=2
  DoorLockIND : Inport  Port=3
  HoodSW : Inport  Port=4
  PsDoorSW : Inport  Port=5
  RLDoorSW : Inport  Port=6
  RRDoorSW : Inport  Port=7
  Tailgate_SW : Inport  Port=8
  BitwiseOR : simulink/Logic and Bit Operations/Bitwise Operator  logicop=OR  UseBitMask=off  NumInputPorts=8  BitMask=bin2dec('11011001')  BitMaskRealWorld=Stored Integer
  SignalPack : FVT_lib/hal/SignalPack  RightShiftCnt=0  BitMask=2^1-1  LeftShiftCnt=3
  SignalPack1 : FVT_lib/hal/SignalPack  RightShiftCnt=0  BitMask=2^1-1  LeftShiftCnt=7
  SignalPack2 : FVT_lib/hal/SignalPack  RightShiftCnt=0  BitMask=2^1-1  LeftShiftCnt=4
  SignalPack3 : FVT_lib/hal/SignalPack  RightShiftCnt=0  BitMask=2^1-1  LeftShiftCnt=5
  SignalPack4 : FVT_lib/hal/SignalPack  RightShiftCnt=0  BitMask=2^1-1  LeftShiftCnt=0
  SignalPack5 : FVT_lib/hal/SignalPack  RightShiftCnt=0  BitMask=2^1-1  LeftShiftCnt=1
  SignalPack6 : FVT_lib/hal/SignalPack  RightShiftCnt=0  BitMask=2^1-1  LeftShiftCnt=2
  SignalPack7 : FVT_lib/hal/SignalPack  RightShiftCnt=0  BitMask=2^1-1  LeftShiftCnt=6
  UnitConverter{,1..15} (16 alike) : DataTypeConversion  OutDataTypeStr=uint8  RndMeth=Round
  Byte_19 : Outport
  wires:
  BitwiseOR/1 -> Byte_19/1
  UnitConverter/1 -> BitwiseOR/1
  SignalPack/1 -> UnitConverter/1
  UnitConverter1/1 -> SignalPack/1
  AllDoorSW/1 -> UnitConverter1/1
  UnitConverter2/1 -> BitwiseOR/2
  SignalPack1/1 -> UnitConverter2/1
  UnitConverter3/1 -> SignalPack1/1
  CTDCtrl/1 -> UnitConverter3/1
  UnitConverter4/1 -> BitwiseOR/3
  SignalPack2/1 -> UnitConverter4/1
  UnitConverter5/1 -> SignalPack2/1
  DoorLockIND/1 -> UnitConverter5/1
  UnitConverter6/1 -> BitwiseOR/4
  SignalPack3/1 -> UnitConverter6/1
  UnitConverter7/1 -> SignalPack3/1
  HoodSW/1 -> UnitConverter7/1
  UnitConverter8/1 -> BitwiseOR/5
  SignalPack4/1 -> UnitConverter8/1
  UnitConverter9/1 -> SignalPack4/1
  PsDoorSW/1 -> UnitConverter9/1
  UnitConverter10/1 -> BitwiseOR/6
  SignalPack5/1 -> UnitConverter10/1
  UnitConverter11/1 -> SignalPack5/1
  RLDoorSW/1 -> UnitConverter11/1
  UnitConverter12/1 -> BitwiseOR/7
  SignalPack6/1 -> UnitConverter12/1
  UnitConverter13/1 -> SignalPack6/1
  RRDoorSW/1 -> UnitConverter13/1
  UnitConverter14/1 -> BitwiseOR/8
  SignalPack7/1 -> UnitConverter14/1
  UnitConverter15/1 -> SignalPack7/1
  Tailgate_SW/1 -> UnitConverter15/1

== system halout/HAL_OUT/CAN4/FD_VCU1_0x116/Byte_2 ==
  CC_Crl_Sta : Inport
  Dr_SeatSta : Inport  Port=2
  MSA_Crl_Sta : Inport  Port=3
  BitwiseOR : simulink/Logic and Bit Operations/Bitwise Operator  logicop=OR  UseBitMask=off  NumInputPorts=3  BitMask=bin2dec('11011001')  BitMaskRealWorld=Stored Integer
  SignalPack : FVT_lib/hal/SignalPack  RightShiftCnt=0  BitMask=2^3-1  LeftShiftCnt=0
  SignalPack1 : FVT_lib/hal/SignalPack  RightShiftCnt=0  BitMask=2^2-1  LeftShiftCnt=6
  SignalPack2 : FVT_lib/hal/SignalPack  RightShiftCnt=0  BitMask=2^3-1  LeftShiftCnt=3
  UnitConverter{,1..5} (6 alike) : DataTypeConversion  OutDataTypeStr=uint8  RndMeth=Round
  Byte_2 : Outport
  wires:
  BitwiseOR/1 -> Byte_2/1
  UnitConverter/1 -> BitwiseOR/1
  SignalPack/1 -> UnitConverter/1
  UnitConverter1/1 -> SignalPack/1
  CC_Crl_Sta/1 -> UnitConverter1/1
  UnitConverter2/1 -> BitwiseOR/2
  SignalPack1/1 -> UnitConverter2/1
  UnitConverter3/1 -> SignalPack1/1
  Dr_SeatSta/1 -> UnitConverter3/1
  UnitConverter4/1 -> BitwiseOR/3
  SignalPack2/1 -> UnitConverter4/1
  UnitConverter5/1 -> SignalPack2/1
  MSA_Crl_Sta/1 -> UnitConverter5/1

== system halout/HAL_OUT/CAN4/FD_VCU1_0x116/Byte_20 ==
  DrDoorSW : Inport
  FD_TBOX_VehData_Err : Inport  Port=2
  FD_TBOX_VehData_Sta : Inport  Port=3
  BitwiseOR : simulink/Logic and Bit Operations/Bitwise Operator  logicop=OR  UseBitMask=off  NumInputPorts=3  BitMask=bin2dec('11011001')  BitMaskRealWorld=Stored Integer
  SignalPack : FVT_lib/hal/SignalPack  RightShiftCnt=0  BitMask=2^1-1  LeftShiftCnt=7
  SignalPack1 : FVT_lib/hal/SignalPack  RightShiftCnt=1  BitMask=2^3-1  LeftShiftCnt=0
  SignalPack2 : FVT_lib/hal/SignalPack  RightShiftCnt=0  BitMask=2^4-1  LeftShiftCnt=3
  UnitConverter{,1..5} (6 alike) : DataTypeConversion  OutDataTypeStr=uint8  RndMeth=Round
  Byte_20 : Outport
  wires:
  BitwiseOR/1 -> Byte_20/1
  UnitConverter/1 -> BitwiseOR/1
  SignalPack/1 -> UnitConverter/1
  UnitConverter1/1 -> SignalPack/1
  DrDoorSW/1 -> UnitConverter1/1
  UnitConverter2/1 -> BitwiseOR/2
  SignalPack1/1 -> UnitConverter2/1
  UnitConverter3/1 -> SignalPack1/1
  FD_TBOX_VehData_Err/1 -> UnitConverter3/1
  UnitConverter4/1 -> BitwiseOR/3
  SignalPack2/1 -> UnitConverter4/1
  UnitConverter5/1 -> SignalPack2/1
  FD_TBOX_VehData_Sta/1 -> UnitConverter5/1

== system halout/HAL_OUT/CAN4/FD_VCU1_0x116/Byte_21 ==
  FD_DKC_VehData_Err : Inport
  FD_DKC_VehData_Sta : Inport  Port=2
  FD_TBOX_VehData_Err : Inport  Port=3
  BitwiseOR : simulink/Logic and Bit Operations/Bitwise Operator  logicop=OR  UseBitMask=off  NumInputPorts=3  BitMask=bin2dec('11011001')  BitMaskRealWorld=Stored Integer
  SignalPack : FVT_lib/hal/SignalPack  RightShiftCnt=1  BitMask=2^3-1  LeftShiftCnt=0
  SignalPack1 : FVT_lib/hal/SignalPack  RightShiftCnt=0  BitMask=2^4-1  LeftShiftCnt=3
  SignalPack2 : FVT_lib/hal/SignalPack  RightShiftCnt=0  BitMask=2^1-1  LeftShiftCnt=7
  UnitConverter{,1..5} (6 alike) : DataTypeConversion  OutDataTypeStr=uint8  RndMeth=Round
  Byte_21 : Outport
  wires:
  BitwiseOR/1 -> Byte_21/1
  UnitConverter/1 -> BitwiseOR/1
  SignalPack/1 -> UnitConverter/1
  UnitConverter1/1 -> SignalPack/1
  FD_DKC_VehData_Err/1 -> UnitConverter1/1
  UnitConverter2/1 -> BitwiseOR/2
  SignalPack1/1 -> UnitConverter2/1
  UnitConverter3/1 -> SignalPack1/1
  FD_DKC_VehData_Sta/1 -> UnitConverter3/1
  UnitConverter4/1 -> BitwiseOR/3
  SignalPack2/1 -> UnitConverter4/1
  UnitConverter5/1 -> SignalPack2/1
  FD_TBOX_VehData_Err/1 -> UnitConverter5/1

== system halout/HAL_OUT/CAN4/FD_VCU1_0x116/Byte_22 ==
  FD_DKC_VehData_Err : Inport
  FD_TBOX_DTCData_Err : Inport  Port=2
  FD_TBOX_DTCData_Sta : Inport  Port=3
  BitwiseOR : simulink/Logic and Bit Operations/Bitwise Operator  logicop=OR  UseBitMask=off  NumInputPorts=3  BitMask=bin2dec('11011001')  BitMaskRealWorld=Stored Integer
  SignalPack : FVT_lib/hal/SignalPack  RightShiftCnt=0  BitMask=2^1-1  LeftShiftCnt=7
  SignalPack1 : FVT_lib/hal/SignalPack  RightShiftCnt=1  BitMask=2^3-1  LeftShiftCnt=0
  SignalPack2 : FVT_lib/hal/SignalPack  RightShiftCnt=0  BitMask=2^4-1  LeftShiftCnt=3
  UnitConverter{,1..5} (6 alike) : DataTypeConversion  OutDataTypeStr=uint8  RndMeth=Round
  Byte_22 : Outport
  wires:
  BitwiseOR/1 -> Byte_22/1
  UnitConverter/1 -> BitwiseOR/1
  SignalPack/1 -> UnitConverter/1
  UnitConverter1/1 -> SignalPack/1
  FD_DKC_VehData_Err/1 -> UnitConverter1/1
  UnitConverter2/1 -> BitwiseOR/2
  SignalPack1/1 -> UnitConverter2/1
  UnitConverter3/1 -> SignalPack1/1
  FD_TBOX_DTCData_Err/1 -> UnitConverter3/1
  UnitConverter4/1 -> BitwiseOR/3
  SignalPack2/1 -> UnitConverter4/1
  UnitConverter5/1 -> SignalPack2/1
  FD_TBOX_DTCData_Sta/1 -> UnitConverter5/1

== system halout/HAL_OUT/CAN4/FD_VCU1_0x116/Byte_23 ==
  AmbLightBreath1 : Inport
  AmbLightBreath2 : Inport  Port=2
  AmbLightBreath3 : Inport  Port=3
  DKCAuthSta : Inport  Port=4
  FD_TBOX_DTCData_Err : Inport  Port=5
  LampPwr : Inport  Port=6
  BitwiseOR : simulink/Logic and Bit Operations/Bitwise Operator  logicop=OR  UseBitMask=off  NumInputPorts=6  BitMask=bin2dec('11011001')  BitMaskRealWorld=Stored Integer
  SignalPack : FVT_lib/hal/SignalPack  RightShiftCnt=0  BitMask=2^1-1  LeftShiftCnt=3
  SignalPack1 : FVT_lib/hal/SignalPack  RightShiftCnt=0  BitMask=2^1-1  LeftShiftCnt=5
  SignalPack2 : FVT_lib/hal/SignalPack  RightShiftCnt=0  BitMask=2^1-1  LeftShiftCnt=6
  SignalPack3 : FVT_lib/hal/SignalPack  RightShiftCnt=0  BitMask=2^2-1  LeftShiftCnt=0
  SignalPack4 : FVT_lib/hal/SignalPack  RightShiftCnt=0  BitMask=2^1-1  LeftShiftCnt=7
  SignalPack5 : FVT_lib/hal/SignalPack  RightShiftCnt=0  BitMask=2^1-1  LeftShiftCnt=4
  UnitConverter{,1..11} (12 alike) : DataTypeConversion  OutDataTypeStr=uint8  RndMeth=Round
  Byte_23 : Outport
  wires:
  BitwiseOR/1 -> Byte_23/1
  UnitConverter/1 -> BitwiseOR/1
  SignalPack/1 -> UnitConverter/1
  UnitConverter1/1 -> SignalPack/1
  AmbLightBreath1/1 -> UnitConverter1/1
  UnitConverter2/1 -> BitwiseOR/2
  SignalPack1/1 -> UnitConverter2/1
  UnitConverter3/1 -> SignalPack1/1
  AmbLightBreath2/1 -> UnitConverter3/1
  UnitConverter4/1 -> BitwiseOR/3
  SignalPack2/1 -> UnitConverter4/1
  UnitConverter5/1 -> SignalPack2/1
  AmbLightBreath3/1 -> UnitConverter5/1
  UnitConverter6/1 -> BitwiseOR/4
  SignalPack3/1 -> UnitConverter6/1
  UnitConverter7/1 -> SignalPack3/1
  DKCAuthSta/1 -> UnitConverter7/1
  UnitConverter8/1 -> BitwiseOR/5
  SignalPack4/1 -> UnitConverter8/1
  UnitConverter9/1 -> SignalPack4/1
  FD_TBOX_DTCData_Err/1 -> UnitConverter9/1
  UnitConverter10/1 -> BitwiseOR/6
  SignalPack5/1 -> UnitConverter10/1
  UnitConverter11/1 -> SignalPack5/1
  LampPwr/1 -> UnitConverter11/1

== system halout/HAL_OUT/CAN4/FD_VCU1_0x116/Byte_24 ==
  AmbLightColor3 : Inport
  BitwiseOR : simulink/Logic and Bit Operations/Bitwise Operator  logicop=OR  UseBitMask=off  BitMask=bin2dec('11011001')  BitMaskRealWorld=Stored Integer
  SignalPack : FVT_lib/hal/SignalPack  RightShiftCnt=0  BitMask=2^6-1  LeftShiftCnt=0
  UnitConverter : DataTypeConversion  OutDataTypeStr=uint8  RndMeth=Round
  UnitConverter1 : DataTypeConversion  OutDataTypeStr=uint8  RndMeth=Round
  Byte_24 : Outport
  wires:
  BitwiseOR/1 -> Byte_24/1
  UnitConverter/1 -> BitwiseOR/1
  SignalPack/1 -> UnitConverter/1
  UnitConverter1/1 -> SignalPack/1
  AmbLightColor3/1 -> UnitConverter1/1

== system halout/HAL_OUT/CAN4/FD_VCU1_0x116/Byte_25 ==
  AmbLightColor2 : Inport
  HWResetSta : Inport  Port=2
  BitwiseOR : simulink/Logic and Bit Operations/Bitwise Operator  logicop=OR  UseBitMask=off  NumInputPorts=2  BitMask=bin2dec('11011001')  BitMaskRealWorld=Stored Integer
  SignalPack : FVT_lib/hal/SignalPack  RightShiftCnt=0  BitMask=2^6-1  LeftShiftCnt=0
  SignalPack1 : FVT_lib/hal/SignalPack  RightShiftCnt=0  BitMask=2^2-1  LeftShiftCnt=6
  UnitConverter{,1..3} (4 alike) : DataTypeConversion  OutDataTypeStr=uint8  RndMeth=Round
  Byte_25 : Outport
  wires:
  BitwiseOR/1 -> Byte_25/1
  UnitConverter/1 -> BitwiseOR/1
  SignalPack/1 -> UnitConverter/1
  UnitConverter1/1 -> SignalPack/1
  AmbLightColor2/1 -> UnitConverter1/1
  UnitConverter2/1 -> BitwiseOR/2
  SignalPack1/1 -> UnitConverter2/1
  UnitConverter3/1 -> SignalPack1/1
  HWResetSta/1 -> UnitConverter3/1

== system halout/HAL_OUT/CAN4/FD_VCU1_0x116/Byte_26 ==
  AmbLightColor1 : Inport
  CtrlDrPwrStbA2 : Inport  Port=2
  CtrlFrPwrStbA1P : Inport  Port=3
  BitwiseOR : simulink/Logic and Bit Operations/Bitwise Operator  logicop=OR  UseBitMask=off  NumInputPorts=3  BitMask=bin2dec('11011001')  BitMaskRealWorld=Stored Integer
  SignalPack : FVT_lib/hal/SignalPack  RightShiftCnt=0  BitMask=2^6-1  LeftShiftCnt=0
  SignalPack1 : FVT_lib/hal/SignalPack  RightShiftCnt=0  BitMask=2^1-1  LeftShiftCnt=6
  SignalPack2 : FVT_lib/hal/SignalPack  RightShiftCnt=0  BitMask=2^1-1  LeftShiftCnt=7
  UnitConverter{,1..5} (6 alike) : DataTypeConversion  OutDataTypeStr=uint8  RndMeth=Round
  Byte_26 : Outport
  wires:
  BitwiseOR/1 -> Byte_26/1
  UnitConverter/1 -> BitwiseOR/1
  SignalPack/1 -> UnitConverter/1
  UnitConverter1/1 -> SignalPack/1
  AmbLightColor1/1 -> UnitConverter1/1
  UnitConverter2/1 -> BitwiseOR/2
  SignalPack1/1 -> UnitConverter2/1
  UnitConverter3/1 -> SignalPack1/1
  CtrlDrPwrStbA2/1 -> UnitConverter3/1
  UnitConverter4/1 -> BitwiseOR/3
  SignalPack2/1 -> UnitConverter4/1
  UnitConverter5/1 -> SignalPack2/1
  CtrlFrPwrStbA1P/1 -> UnitConverter5/1

== system halout/HAL_OUT/CAN4/FD_VCU1_0x116/Byte_27 ==
  AmbLightBrightness3 : Inport
  CtrlFrIRC1 : Inport  Port=2
  BitwiseOR : simulink/Logic and Bit Operations/Bitwise Operator  logicop=OR  UseBitMask=off  NumInputPorts=2  BitMask=bin2dec('11011001')  BitMaskRealWorld=Stored Integer
  SignalPack : FVT_lib/hal/SignalPack  RightShiftCnt=0  BitMask=2^7-1  LeftShiftCnt=0
  SignalPack1 : FVT_lib/hal/SignalPack  RightShiftCnt=0  BitMask=2^1-1  LeftShiftCnt=7
  UnitConverter{,1..3} (4 alike) : DataTypeConversion  OutDataTypeStr=uint8  RndMeth=Round
  Byte_27 : Outport
  wires:
  BitwiseOR/1 -> Byte_27/1
  UnitConverter/1 -> BitwiseOR/1
  SignalPack/1 -> UnitConverter/1
  UnitConverter1/1 -> SignalPack/1
  AmbLightBrightness3/1 -> UnitConverter1/1
  UnitConverter2/1 -> BitwiseOR/2
  SignalPack1/1 -> UnitConverter2/1
  UnitConverter3/1 -> SignalPack1/1
  CtrlFrIRC1/1 -> UnitConverter3/1

== system halout/HAL_OUT/CAN4/FD_VCU1_0x116/Byte_28 ==
  AmbLightBrightness2 : Inport
  CtrlFrEDUINVERTER : Inport  Port=2
  BitwiseOR : simulink/Logic and Bit Operations/Bitwise Operator  logicop=OR  UseBitMask=off  NumInputPorts=2  BitMask=bin2dec('11011001')  BitMaskRealWorld=Stored Integer
  SignalPack : FVT_lib/hal/SignalPack  RightShiftCnt=0  BitMask=2^7-1  LeftShiftCnt=0
  SignalPack1 : FVT_lib/hal/SignalPack  RightShiftCnt=0  BitMask=2^1-1  LeftShiftCnt=7
  UnitConverter{,1..3} (4 alike) : DataTypeConversion  OutDataTypeStr=uint8  RndMeth=Round
  Byte_28 : Outport
  wires:
  BitwiseOR/1 -> Byte_28/1
  UnitConverter/1 -> BitwiseOR/1
  SignalPack/1 -> UnitConverter/1
  UnitConverter1/1 -> SignalPack/1
  AmbLightBrightness2/1 -> UnitConverter1/1
  UnitConverter2/1 -> BitwiseOR/2
  SignalPack1/1 -> UnitConverter2/1
  UnitConverter3/1 -> SignalPack1/1
  CtrlFrEDUINVERTER/1 -> UnitConverter3/1

== system halout/HAL_OUT/CAN4/FD_VCU1_0x116/Byte_29 ==
  AmbLightBrightness1 : Inport
  CtrlFrBMSCCUCIR : Inport  Port=2
  BitwiseOR : simulink/Logic and Bit Operations/Bitwise Operator  logicop=OR  UseBitMask=off  NumInputPorts=2  BitMask=bin2dec('11011001')  BitMaskRealWorld=Stored Integer
  SignalPack : FVT_lib/hal/SignalPack  RightShiftCnt=0  BitMask=2^7-1  LeftShiftCnt=0
  SignalPack1 : FVT_lib/hal/SignalPack  RightShiftCnt=0  BitMask=2^1-1  LeftShiftCnt=7
  UnitConverter{,1..3} (4 alike) : DataTypeConversion  OutDataTypeStr=uint8  RndMeth=Round
  Byte_29 : Outport
  wires:
  BitwiseOR/1 -> Byte_29/1
  UnitConverter/1 -> BitwiseOR/1
  SignalPack/1 -> UnitConverter/1
  UnitConverter1/1 -> SignalPack/1
  AmbLightBrightness1/1 -> UnitConverter1/1
  UnitConverter2/1 -> BitwiseOR/2
  SignalPack1/1 -> UnitConverter2/1
  UnitConverter3/1 -> SignalPack1/1
  CtrlFrBMSCCUCIR/1 -> UnitConverter3/1

== system halout/HAL_OUT/CAN4/FD_VCU1_0x116/Byte_3 ==
  PwrSta : Inport
  ReBrakeLPReq : Inport  Port=2
  ShiftGearPosn : Inport  Port=3
  BitwiseOR : simulink/Logic and Bit Operations/Bitwise Operator  logicop=OR  UseBitMask=off  NumInputPorts=3  BitMask=bin2dec('11011001')  BitMaskRealWorld=Stored Integer
  SignalPack : FVT_lib/hal/SignalPack  RightShiftCnt=0  BitMask=2^3-1  LeftShiftCnt=2
  SignalPack1 : FVT_lib/hal/SignalPack  RightShiftCnt=0  BitMask=2^1-1  LeftShiftCnt=1
  SignalPack2 : FVT_lib/hal/SignalPack  RightShiftCnt=0  BitMask=2^3-1  LeftShiftCnt=5
  UnitConverter{,1..5} (6 alike) : DataTypeConversion  OutDataTypeStr=uint8  RndMeth=Round
  Byte_3 : Outport
  wires:
  BitwiseOR/1 -> Byte_3/1
  UnitConverter/1 -> BitwiseOR/1
  SignalPack/1 -> UnitConverter/1
  UnitConverter1/1 -> SignalPack/1
  PwrSta/1 -> UnitConverter1/1
  UnitConverter2/1 -> BitwiseOR/2
  SignalPack1/1 -> UnitConverter2/1
  UnitConverter3/1 -> SignalPack1/1
  ReBrakeLPReq/1 -> UnitConverter3/1
  UnitConverter4/1 -> BitwiseOR/3
  SignalPack2/1 -> UnitConverter4/1
  UnitConverter5/1 -> SignalPack2/1
  ShiftGearPosn/1 -> UnitConverter5/1

== system halout/HAL_OUT/CAN4/FD_VCU1_0x116/Byte_30 ==
  VehSpeed : Inport
  BitwiseOR : simulink/Logic and Bit Operations/Bitwise Operator  logicop=OR  UseBitMask=off  BitMask=bin2dec('11011001')  BitMaskRealWorld=Stored Integer
  SignalPack : FVT_lib/hal/SignalPack  RightShiftCnt=8  BitMask=2^4-1  LeftShiftCnt=0
  UnitConverter : DataTypeConversion  OutDataTypeStr=uint8  RndMeth=Round
  UnitConverter1 : DataTypeConversion  OutDataTypeStr=uint16  RndMeth=Round
  convert_out : FVT_lib/hal/convert_out  gain=0.125  offset=0
  Byte_30 : Outport
  wires:
  BitwiseOR/1 -> Byte_30/1
  UnitConverter/1 -> BitwiseOR/1
  SignalPack/1 -> UnitConverter/1
  UnitConverter1/1 -> SignalPack/1
  convert_out/1 -> UnitConverter1/1
  VehSpeed/1 -> convert_out/1

== system halout/HAL_OUT/CAN4/FD_VCU1_0x116/Byte_31 ==
  VehSpeed : Inport
  BitwiseOR : simulink/Logic and Bit Operations/Bitwise Operator  logicop=OR  UseBitMask=off  BitMask=bin2dec('11011001')  BitMaskRealWorld=Stored Integer
  SignalPack : FVT_lib/hal/SignalPack  RightShiftCnt=0  BitMask=2^8-1  LeftShiftCnt=0
  UnitConverter : DataTypeConversion  OutDataTypeStr=uint8  RndMeth=Round
  UnitConverter1 : DataTypeConversion  OutDataTypeStr=uint16  RndMeth=Round
  convert_out : FVT_lib/hal/convert_out  gain=0.125  offset=0
  Byte_31 : Outport
  wires:
  BitwiseOR/1 -> Byte_31/1
  UnitConverter/1 -> BitwiseOR/1
  SignalPack/1 -> UnitConverter/1
  UnitConverter1/1 -> SignalPack/1
  convert_out/1 -> UnitConverter1/1
  VehSpeed/1 -> convert_out/1

== system halout/HAL_OUT/CAN4/FD_VCU1_0x116/Byte_4 ==
  DKCTimeSN : Inport
  BitwiseOR : simulink/Logic and Bit Operations/Bitwise Operator  logicop=OR  UseBitMask=off  BitMask=bin2dec('11011001')  BitMaskRealWorld=Stored Integer
  SignalPack : FVT_lib/hal/SignalPack  RightShiftCnt=24  BitMask=2^8-1  LeftShiftCnt=0
  UnitConverter : DataTypeConversion  OutDataTypeStr=uint8  RndMeth=Round
  UnitConverter1 : DataTypeConversion  OutDataTypeStr=uint32  RndMeth=Round
  Byte_4 : Outport
  wires:
  BitwiseOR/1 -> Byte_4/1
  UnitConverter/1 -> BitwiseOR/1
  SignalPack/1 -> UnitConverter/1
  UnitConverter1/1 -> SignalPack/1
  DKCTimeSN/1 -> UnitConverter1/1

== system halout/HAL_OUT/CAN4/FD_VCU1_0x116/Byte_5 ==
  DKCTimeSN : Inport
  BitwiseOR : simulink/Logic and Bit Operations/Bitwise Operator  logicop=OR  UseBitMask=off  BitMask=bin2dec('11011001')  BitMaskRealWorld=Stored Integer
  SignalPack : FVT_lib/hal/SignalPack  RightShiftCnt=16  BitMask=2^8-1  LeftShiftCnt=0
  UnitConverter : DataTypeConversion  OutDataTypeStr=uint8  RndMeth=Round
  UnitConverter1 : DataTypeConversion  OutDataTypeStr=uint32  RndMeth=Round
  Byte_5 : Outport
  wires:
  BitwiseOR/1 -> Byte_5/1
  UnitConverter/1 -> BitwiseOR/1
  SignalPack/1 -> UnitConverter/1
  UnitConverter1/1 -> SignalPack/1
  DKCTimeSN/1 -> UnitConverter1/1

== system halout/HAL_OUT/CAN4/FD_VCU1_0x116/Byte_6 ==
  DKCTimeSN : Inport
  BitwiseOR : simulink/Logic and Bit Operations/Bitwise Operator  logicop=OR  UseBitMask=off  BitMask=bin2dec('11011001')  BitMaskRealWorld=Stored Integer
  SignalPack : FVT_lib/hal/SignalPack  RightShiftCnt=8  BitMask=2^8-1  LeftShiftCnt=0
  UnitConverter : DataTypeConversion  OutDataTypeStr=uint8  RndMeth=Round
  UnitConverter1 : DataTypeConversion  OutDataTypeStr=uint32  RndMeth=Round
  Byte_6 : Outport
  wires:
  BitwiseOR/1 -> Byte_6/1
  UnitConverter/1 -> BitwiseOR/1
  SignalPack/1 -> UnitConverter/1
  UnitConverter1/1 -> SignalPack/1
  DKCTimeSN/1 -> UnitConverter1/1

== system halout/HAL_OUT/CAN4/FD_VCU1_0x116/Byte_7 ==
  DKCTimeSN : Inport
  BitwiseOR : simulink/Logic and Bit Operations/Bitwise Operator  logicop=OR  UseBitMask=off  BitMask=bin2dec('11011001')  BitMaskRealWorld=Stored Integer
  SignalPack : FVT_lib/hal/SignalPack  RightShiftCnt=0  BitMask=2^8-1  LeftShiftCnt=0
  UnitConverter : DataTypeConversion  OutDataTypeStr=uint8  RndMeth=Round
  UnitConverter1 : DataTypeConversion  OutDataTypeStr=uint32  RndMeth=Round
  Byte_7 : Outport
  wires:
  BitwiseOR/1 -> Byte_7/1
  UnitConverter/1 -> BitwiseOR/1
  SignalPack/1 -> UnitConverter/1
  UnitConverter1/1 -> SignalPack/1
  DKCTimeSN/1 -> UnitConverter1/1

== system halout/HAL_OUT/CAN4/FD_VCU1_0x116/Byte_8 ==
  TimeSNDKCFbk : Inport
  BitwiseOR : simulink/Logic and Bit Operations/Bitwise Operator  logicop=OR  UseBitMask=off  BitMask=bin2dec('11011001')  BitMaskRealWorld=Stored Integer
  SignalPack : FVT_lib/hal/SignalPack  RightShiftCnt=24  BitMask=2^8-1  LeftShiftCnt=0
  UnitConverter : DataTypeConversion  OutDataTypeStr=uint8  RndMeth=Round
  UnitConverter1 : DataTypeConversion  OutDataTypeStr=uint32  RndMeth=Round
  Byte_8 : Outport
  wires:
  BitwiseOR/1 -> Byte_8/1
  UnitConverter/1 -> BitwiseOR/1
  SignalPack/1 -> UnitConverter/1
  UnitConverter1/1 -> SignalPack/1
  TimeSNDKCFbk/1 -> UnitConverter1/1

== system halout/HAL_OUT/CAN4/FD_VCU1_0x116/Byte_9 ==
  TimeSNDKCFbk : Inport
  BitwiseOR : simulink/Logic and Bit Operations/Bitwise Operator  logicop=OR  UseBitMask=off  BitMask=bin2dec('11011001')  BitMaskRealWorld=Stored Integer
  SignalPack : FVT_lib/hal/SignalPack  RightShiftCnt=16  BitMask=2^8-1  LeftShiftCnt=0
  UnitConverter : DataTypeConversion  OutDataTypeStr=uint8  RndMeth=Round
  UnitConverter1 : DataTypeConversion  OutDataTypeStr=uint32  RndMeth=Round
  Byte_9 : Outport
  wires:
  BitwiseOR/1 -> Byte_9/1
  UnitConverter/1 -> BitwiseOR/1
  SignalPack/1 -> UnitConverter/1
  UnitConverter1/1 -> SignalPack/1
  TimeSNDKCFbk/1 -> UnitConverter1/1

== system halout/HAL_OUT/CAN4/FD_VCU1_0x116/CCCrlSta ==
  CCCrlSta : Inport
  Data Type Conversion : DataTypeConversion  OutDataTypeStr=uint8  RndMeth=Round
  CAN4_CC_Crl_Sta : Outport
  wires:
  Data Type Conversion/1 -> CAN4_CC_Crl_Sta/1
  CCCrlSta/1 -> Data Type Conversion/1

== system halout/HAL_OUT/CAN4/FD_VCU1_0x116/CSVCU1CAN4 ==
  CSVCU1CAN4 : Inport
  Data Type Conversion : DataTypeConversion  OutDataTypeStr=uint8  RndMeth=Round
  CAN4_CS_VCU1_CAN4 : Outport
  wires:
  Data Type Conversion/1 -> CAN4_CS_VCU1_CAN4/1
  CSVCU1CAN4/1 -> Data Type Conversion/1

== system halout/HAL_OUT/CAN4/FD_VCU1_0x116/CTDCtrl ==
  CTDCtrl : Inport
  Data Type Conversion : DataTypeConversion  OutDataTypeStr=uint8  RndMeth=Round
  CAN4_CTDCtrl : Outport
  wires:
  Data Type Conversion/1 -> CAN4_CTDCtrl/1
  CTDCtrl/1 -> Data Type Conversion/1

== system halout/HAL_OUT/CAN4/FD_VCU1_0x116/CTDLockSW ==
  CTDLockSW : Inport
  Data Type Conversion : DataTypeConversion  OutDataTypeStr=uint8  RndMeth=Round
  CAN4_CTDLockSW : Outport
  wires:
  Data Type Conversion/1 -> CAN4_CTDLockSW/1
  CTDLockSW/1 -> Data Type Conversion/1

== system halout/HAL_OUT/CAN4/FD_VCU1_0x116/CTDUnlockSW ==
  CTDUnlockSW : Inport
  Data Type Conversion : DataTypeConversion  OutDataTypeStr=uint8  RndMeth=Round
  CAN4_CTDUnlockSW : Outport
  wires:
  Data Type Conversion/1 -> CAN4_CTDUnlockSW/1
  CTDUnlockSW/1 -> Data Type Conversion/1

== system halout/HAL_OUT/CAN4/FD_VCU1_0x116/CrashDetd ==
  CrashDetd : Inport
  Data Type Conversion : DataTypeConversion  OutDataTypeStr=uint8  RndMeth=Round
  CAN4_CrashDetd : Outport
  wires:
  Data Type Conversion/1 -> CAN4_CrashDetd/1
  CrashDetd/1 -> Data Type Conversion/1

== system halout/HAL_OUT/CAN4/FD_VCU1_0x116/CtrlDrPwrStbA2 ==
  CtrlDrPwrStbA2 : Inport
  Data Type Conversion : DataTypeConversion  OutDataTypeStr=uint8  RndMeth=Round
  CAN4_CtrlDrPwrStbA2 : Outport
  wires:
  Data Type Conversion/1 -> CAN4_CtrlDrPwrStbA2/1
  CtrlDrPwrStbA2/1 -> Data Type Conversion/1

== system halout/HAL_OUT/CAN4/FD_VCU1_0x116/CtrlFrBMSCCUCIR ==
  CtrlFrBMSCCUCIR : Inport
  Data Type Conversion : DataTypeConversion  OutDataTypeStr=uint8  RndMeth=Round
  CAN4_CtrlFrBMSCCUCIR : Outport
  wires:
  Data Type Conversion/1 -> CAN4_CtrlFrBMSCCUCIR/1
  CtrlFrBMSCCUCIR/1 -> Data Type Conversion/1

== system halout/HAL_OUT/CAN4/FD_VCU1_0x116/CtrlFrEDUINVERTER ==
  CtrlFrEDUINVERTER : Inport
  Data Type Conversion : DataTypeConversion  OutDataTypeStr=uint8  RndMeth=Round
  CAN4_CtrlFrEDUINVERTER : Outport
  wires:
  Data Type Conversion/1 -> CAN4_CtrlFrEDUINVERTER/1
  CtrlFrEDUINVERTER/1 -> Data Type Conversion/1

== system halout/HAL_OUT/CAN4/FD_VCU1_0x116/CtrlFrIRC1 ==
  CtrlFrIRC1 : Inport
  Data Type Conversion : DataTypeConversion  OutDataTypeStr=uint8  RndMeth=Round
  CAN4_CtrlFrIRC1 : Outport
  wires:
  Data Type Conversion/1 -> CAN4_CtrlFrIRC1/1
  CtrlFrIRC1/1 -> Data Type Conversion/1
